simulink model "bbolpfb14r1"  (R2012b)
settings: Solver=VariableStepDiscrete  SolverMode=SingleTasking  StartTime=0.0  StopTime=10.0  RelTol=1e-3
undefined symbols (not defined in the file or in its folder): pfb_coeff_gen_calc
undefined symbols (not defined in the file): bit_reverse
libraries: xbsIndex_r4 x7954, casper_library_misc x51, casper_library_delays x20, xps_library x5
(part 13 of 103)

== system bbolpfb14r1/fft_biplex_2by2_real/butterfly_direct1/twiddle ==
  ai : Inport
  bi : Inport  Port=2
  sync_in : Inport  Port=3
  bus_convert : Subsystem  AncestorBlock=casper_library_bus/bus_convert  mask(bus_convert){n_bits_in=repmat(input_bit_width+coeff_bit_width+1, 1, n_inputs), bin_pt_in=(bin_pt_in+coeff_bit_width-1), cmplx=on, n_bits_out=input_bit_width+1, bin_pt_out=bin_pt_in, quantization=0, overflow=0, latency=conv_latency, of=off, misc=on}
      mask prompts: n_bits_in "input bit widths"; bin_pt_in "input binary points"; cmplx "input complex"; n_bits_out "output bit widths"; bin_pt_out "output binary points"; quantization "quantization strategy (Truncate=0, Round  (unbiased: +/- Inf)=1, Round (unbiased: Even Values)=2)"; overflow "overflow strategy (Wrap=0, Saturate=1, Flag as error=2)"; of "overflow indication"; misc "misc support"
      mask help: Convert components of busses
      mask init: same as bbolpfb14r1/fft_biplex_2by2_real/butterfly_direct1/bus_convert
  bus_create : Subsystem  AncestorBlock=casper_library_flow_control/bus_create  mask(bus_create){inputNum=3}
      mask prompts: inputNum "Number of inputs:"
      mask init:
      | bus_create_init(gcb,...
      |     'inputNum', inputNum);
  bus_expand : Subsystem  AncestorBlock=casper_library_flow_control/bus_expand  mask(bus_expand){mode=divisions of arbitrary size, outputNum=1, outputWidth=[n_inputs*input_bit_width*2, 1+(n_inputs*input_bit_width*2)], outputBinaryPt=[0 0], outputArithmeticType=[0 0], show_format=off, outputToWorkspace=off, variablePrefix=out, outputToModelAsWell=on}
      mask prompts: outputNum "Number of outputs:"; outputWidth "Output width [msb ... lsb]:"; outputBinaryPt "Output binary point position [msb ... lsb]:"; outputArithmeticType "Output arithmetic type (ufix=0, fix=1, bool=2) [msb ... lsb]:"; show_format "Print format string?"; outputToWorkspace "Output to workspace?"; variablePrefix "Variable name prefix:"; outputToModelAsWell "Output to model as well?"
      mask help:
      | Expands a 'bus' made using a bus_create or Xilinx
      | concat block.
      | The input will be divided into the specified number
      | of outputs with the specified arithmetic types.
      | Divisions are made from most significant bit.
      mask init: same as bbolpfb14r1/bus_expand
      settings: AttributesFormatString=2 outputs
      mask TypeOptions mode: divisions of equal size | divisions of arbitrary size
      mask Callback mode: bus_expand_callback();
      mask Callback outputWidth: bus_expand_callback();
      mask Callback outputToWorkspace: bus_expand_callback();
  bus_expand1 : Subsystem  AncestorBlock=casper_library_flow_control/bus_expand  mask(bus_expand){mode=divisions of arbitrary size, outputNum=1, outputWidth=[1 36], outputBinaryPt=[0 0], outputArithmeticType=[2 0], show_format=off, outputToWorkspace=off, variablePrefix=out, outputToModelAsWell=on}
      mask prompts: outputNum "Number of outputs:"; outputWidth "Output width [msb ... lsb]:"; outputBinaryPt "Output binary point position [msb ... lsb]:"; outputArithmeticType "Output arithmetic type (ufix=0, fix=1, bool=2) [msb ... lsb]:"; show_format "Print format string?"; outputToWorkspace "Output to workspace?"; variablePrefix "Variable name prefix:"; outputToModelAsWell "Output to model as well?"
      mask help:
      | Expands a 'bus' made using a bus_create or Xilinx
      | concat block.
      | The input will be divided into the specified number
      | of outputs with the specified arithmetic types.
      | Divisions are made from most significant bit.
      mask init: same as bbolpfb14r1/bus_expand
      settings: AttributesFormatString=2 outputs
      mask TypeOptions mode: divisions of equal size | divisions of arbitrary size
      mask Callback mode: bus_expand_callback();
      mask Callback outputWidth: bus_expand_callback();
      mask Callback outputToWorkspace: bus_expand_callback();
  bus_mult : Subsystem  AncestorBlock=casper_library_bus/bus_mult  mask(bus_mult){n_bits_a=coeff_bit_width, bin_pt_a=coeff_bit_width-1, type_a=1, cmplx_a=on, n_bits_b=18, bin_pt_b=bin_pt_in, type_b=1, cmplx_b=on, n_bits_out=input_bit_width+coeff_bit_width+1, bin_pt_out=(bin_pt_in+coeff_bit_width-1), type_out=1, quantization=0, overflow=0, mult_latency=mult_latency, add_latency=add_latency, conv_latency=0, max_fanout=max_fanout, fan_latency=1, multiplier_implementation=behavioral HDL, misc=on}
      mask prompts: n_bits_a "a input bit widths"; bin_pt_a "a input binary points"; type_a "a input type (Unsigned=0, Signed=1)"; cmplx_a "a input complex"; n_bits_b "b input bit widths"; bin_pt_b "b input binary points"; type_b "b input type (Unsigned=0, Signed=1)"; cmplx_b "b input complex"; n_bits_out "output bit widths"; bin_pt_out "output binary points"; type_out "output type (Unsigned=0, Signed=1)"; quantization "quantization strategy (Truncate=0, Round  (unbiased: +/- Inf)=1)"; overflow "overflow strategy (Wrap=0, Saturate=1, Flag as error=2)"; mult_latency "multiplier latency"; add_latency "adder latency"; conv_latency "convert latency"; max_fanout "limit fanout to ?"; fan_latency "fanout register latency"; multiplier_implementation "multiplier implementation"; misc "misc support"
      mask help: Multiply components of two busses
      mask init:
      | bus_mult_init(gcb, ...
      |     'n_bits_a', n_bits_a, ...
      |     'bin_pt_a', bin_pt_a, ...
      |     'type_a', type_a, ...
      |     'cmplx_a', cmplx_a, ...
      |     'n_bits_b', n_bits_b, ...
      |     'bin_pt_b', bin_pt_b, ...
      |     'type_b', type_b, ...
      |     'cmplx_b', cmplx_b, ...
      |     'n_bits_out', n_bits_out, ...
      |     'bin_pt_out', bin_pt_out, ...
      |     'type_out', type_out, ...
      |     'quantization', quantization, ...
      |     'overflow', overflow, ...
      |     'mult_latency', mult_latency, ...
      |     'add_latency', add_latency, ...
      |     'conv_latency', conv_latency, ...
      |     'max_fanout', max_fanout, ...
      |     'fan_latency', fan_latency, ...
      |     'multiplier_implementation', multiplier_implementation, ...
      |     'misc', misc);
      mask TypeOptions multiplier_implementation: behavioral HDL | standard core | embedded multiplier core
  coeff_gen : Subsystem  AncestorBlock=casper_library_ffts_twiddle_coeff_gen/coeff_gen  mask(coeff_gen){FFTSize=FFTSize, Coeffs=[0 8192 4096 12288 2048 10240 6144 14336 1024 9216 5120 13312 3072 11264 7168 15360 512 8704 4608 12800 2560 10752 6656 14848 1536 9728 5632 13824 3584 11776 7680 15872 256 8448 4352 12544 2304 10496 6400 14592 1280 9472 5376 13568 3328 11520 7424 15616 768 8960 4864 13056 2816 11008 6912 15104 1792 9984 5888 14080 3840 12032 7936 16128 128 8320 4224 12416 2176 10368 6272 14464 1152 9344 5248 13440 3200 11392 7296 15488 640 8832 4736 12928 2688 10880 6784 14976 1664 9856 5760 13952 3712 11904 7808 16000 384 8576 4480 12672 2432 10624 6528 14720 1408 9600 5504 13696 3456 11648 7552 15744 896 9088 4992 13184 2944 11136 7040 15232 1920 10112 6016 14208 3968 12160 8064 16256 64 8256 4160 12352 2112 10304 6208 14400 1088 9280 5184 13376 3136 11328 7232 15424 576 8768 4672 12864 2624 10816 6720 14912 1600 9792 5696 13888 3648 11840 7744 15936 320 8512 4416 12608 2368 10560 6464 14656 1344 9536 5440 13632 3392 11584 7488 15680 832 9024 4928 13120 2880 11072 6976 15168 1856 10048 5952 14144 3904 12096 8000 16192 192 8384 4288 12480 2240 10432 6336 14528 1216 9408 5312 13504 3264 11456 7360 15552 704 8896 4800 12992 2752 10944 6848 15040 1728 9920 5824 14016 3776 11968 7872 16064 448 8640 4544 12736 2496 10688 6592 14784 1472 9664 5568 13760 3520 11712 7616 15808 960 9152 5056 13248 3008 11200 7104 15296 1984 10176 6080 14272 4032 12224 8128 16320 32 8224 4128 12320 2080 10272 6176 14368 1056 9248 5152 13344 3104 11296 7200 15392 544 8736 4640 12832 2592 10784 6688 14880 1568 9760 5664 13856 3616 11808 7712 15904 288 8480 4384 12576 2336 10528 6432 14624 1312 9504 5408 13600 3360 11552 7456 15648 800 8992 4896 13088 2848 11040 6944 15136 1824 10016 5920 14112 3872 12064 7968 16160 160 8352 4256 12448 2208 10400 6304 14496 1184 9376 5280 13472 3232 11424 7328 15520 672 8864 4768 12960 2720 10912 6816 15008 1696 9888 5792 13984 3744 11936 7840 16032 416 8608 4512 12704 2464 10656 6560 14752 1440 9632 5536 13728 3488 11680 7584 15776 928 9120 5024 13216 2976 11168 7072 15264 1952 10144 6048 14240 4000 12192 8096 16288 96 8288 4192 12384 2144 10336 6240 14432 1120 9312 5216 13408 3168 11360 7264 15456 608 8800 4704 12896 2656 10848 6752 14944 1632 9824 5728 13920 3680 11872 7776 15968 352 8544 4448 12640 2400 10592 6496 14688 1376 9568 5472 13664 3424 11616 7520 15712 864 9056 4960 13152 2912 11104 7008 15200 1888 10080 5984 14176 3936 12128 8032 16224 224 8416 4320 12512 2272 10464 6368 14560 1248 9440 5344 13536 3296 11488 7392 15584 736 8928 4832 13024 2784 10976 6880 15072 1760 9952 5856 14048 3808 12000 7904 16096 480 8672 4576 12768 2528 10720 6624 14816 1504 9696 5600 13792 3552 11744 7648 15840 992 9184 5088 13280 3040 11232 7136 15328 2016 10208 6112 14304 4064 12256 8160 16352 16 8208 4112 12304 2064 10256 6160 14352 1040 9232 5136 13328 3088 11280 7184 15376 528 8720 4624 12816 2576 10768 6672 14864 1552 9744 5648 13840 3600 11792 7696 15888 272 8464 4368 12560 2320 10512 6416 14608 1296 9488 5392 13584 3344 11536 7440 15632 784 8976 4880 13072 2832 11024 6928 15120 1808 10000 5904 14096 3856 12048 7952 16144 144 8336 4240 12432 2192 10384 6288 14480 1168 9360 5264 13456 3216 11408 7312 15504 656 8848 4752 12944 2704 10896 6800 14992 1680 9872 5776 13968 3728 11920 7824 16016 400 8592 4496 12688 2448 10640 6544 14736 1424 9616 5520 13712 3472 11664 7568 15760 912 9104 5008 13200 2960 11152 7056 15248 1936 10128 6032 14224 3984 12176 8080 16272 80 8272 4176 12368 2128 10320 6224 14416 1104 9296 5200 13392 3152 11344 7248 15440 592 8784 4688 12880 2640 10832 6736 14928 1616 9808 5712 13904 3664 11856 7760 15952 336 8528 4432 12624 2384 10576 6480 14672 1360 9552 5456 13648 3408 11600 7504 15696 848 9040 4944 13136 2896 11088 6992 15184 1872 10064 5968 14160 3920 12112 8016 16208 208 8400 4304 12496 2256 10448 6352 14544 1232 9424 5328 13520 3280 11472 7376 15568 720 8912 4816 13008 2768 10960 6864 15056 1744 9936 5840 14032 3792 11984 7888 16080 464 8656 4560 12752 2512 10704 6608 14800 1488 9680 5584 13776 3536 11728 7632 15824 ...(+83196 chars)], coeff_bit_width=coeff_bit_width, StepPeriod=StepPeriod, async=off, misc=on, bram_latency=bram_latency, mult_latency=mult_latency, add_latency=add_latency, conv_latency=conv_latency, coeffs_bit_limit=coeffs_bit_limit, coeff_sharing=on, coeff_decimation=on, coeff_generation=on, cal_bits=cal_bits, n_bits_rotation=n_bits_rotation, quantization=Truncate}
      mask prompts: FFTSize "fft size (2^?)"; Coeffs "Coefficients"; coeff_bit_width "Coefficient Bit Width:"; StepPeriod "Step Period: (2^?)"; async "asynchronous operation"; misc "misc port"; bram_latency "BRAM latency"; mult_latency "Multiplier latency"; add_latency "Adder latency"; conv_latency "Convert latency"; coeffs_bit_limit "Number bits above which to store stage's coefficients in BRAM (2^? bits)"; coeff_sharing "BRAM sharing in coeff storage"; coeff_decimation "Store a fraction of coeff factors where useful"; coeff_generation "Generate coeffs with multipliers where useful"; cal_bits "Number calibration locations when generating coeffs (2^?)"; n_bits_rotation "Rotation vector resolution"; quantization "Quantization strategy"
      mask help:
      | Generates a sequence of complex coefficients for use in generating twiddle
      | factors for FFTs.
      mask init:
      | coeff_gen_init(gcb, ...
      |    'FFTSize', FFTSize, ...
      |    'Coeffs', Coeffs, ...
      |    'coeff_bit_width', coeff_bit_width, ...
      |    'StepPeriod', StepPeriod, ...
      |    'async', async, ...
      |    'misc', misc, ...
      |    'bram_latency', bram_latency, ...
      |    'mult_latency', mult_latency, ...
      |    'add_latency', add_latency, ...
      |    'conv_latency', conv_latency, ...
      |    'coeffs_bit_limit', coeffs_bit_limit, ...
      |    'coeff_sharing', coeff_sharing, ...
      |    'coeff_decimation', coeff_decimation, ...
      |    'coeff_generation', coeff_generation, ...
      |    'cal_bits', cal_bits, ...
      |    'n_bits_rotation', n_bits_rotation, ...
      |    'quantization', quantization);
      settings: AttributesFormatString=16384 @ (18,17)
      mask TypeOptions quantization: Truncate | Round  (unbiased: +/- Inf) | Round  (unbiased: Even Values)
  ao : Outport
  bwo : Outport  Port=2
  sync_out : Outport  Port=3
  wires:
  bi/1 -> bus_create/1(in1)
  sync_in/1 -> bus_create/2(in2), coeff_gen/1(rst)
  ai/1 -> bus_create/3(in3)
  bus_create/1(bus_out) -> coeff_gen/2(misci)
  coeff_gen/2(misco) -> bus_expand/1(bus_in)
  coeff_gen/1(w) -> bus_mult/1(a)
  bus_expand/2(lsb_out1) -> bus_mult/3(misci)
  bus_expand/1(msb_out2) -> bus_mult/2(b)
  bus_mult/1(a*b) -> bus_convert/1(din)
  bus_mult/2(misco) -> bus_convert/2(misci)
  bus_convert/1(dout) -> bwo/1
  bus_convert/2(misco) -> bus_expand1/1(bus_in)
  bus_expand1/1(msb_out2) -> sync_out/1
  bus_expand1/2(lsb_out1) -> ao/1
